simulink model "light_luminance"  (Simulink 10.0)
settings: Solver=FixedStepAuto  StartTime=0.0  StopTime=60  FixedStep=fixedStep  MaxStep=0.2  RelTol=1e-3
values from neighbouring files (symbols this model uses):
  L0Source1 = 1200    [lightModel.m]
  startLightSource = 0    [lightModel.m]
  timeLightSource = 20    [lightModel.m]
settings Model: Creator=lixuansong  LastModifiedBy=Ozgur Ozmen
settings DataIOCC: SaveFormat=Dataset  ReturnWorkspaceOutputs=on
settings OptimizationCC: LifeSpan=auto
settings DebuggingCC: UnderspecifiedInitializationDetection=Simplified  MergeDetectMultiDrivingBlocksExec=error  SFUnexpectedBacktrackingDiag=error  SFNoUnconditionalDefaultTransitionDiag=error  SFExecutionAtInitializationDiag=warning  ArithmeticOperatorsInVariantConditions=error
settings HardwareCC: ProdBitPerPointer=64  ProdBitPerSizeT=64  ProdBitPerPtrDiffT=64  ProdLargestAtomicFloat=Float  ProdIntDivRoundTo=Zero  ProdEndianess=LittleEndian  ProdWordSize=64  ProdHWDeviceType=Intel->x86-64 (Windows64)
settings ModelReferenceCC: PropagateSignalLabelsOutOfModel=on
settings SFSimCC: SimUseLocalCustomCode=on  CustomCodeUndefinedFunction=FilterOut
settings RTWCC: RTWUseLocalCustomCode=on
settings CodeAppCC: StateflowObjectComments=off
settings GRTTargetCC: TargetLangStandard=C99 (ISO)  CombineOutputUpdateFcns=on  GRTInterface=off
settings ConfigComp: CovMetricSettings=dwe  CovHtmlReporting=off  CovSaveCumulativeToWorkspaceVar=off  CovSaveSingleToWorkspaceVar=off

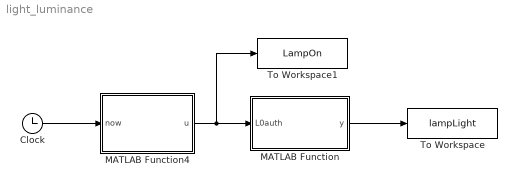
== system light_luminance ==
  Clock : Clock
  MATLAB Function : MATLAB Function  TreatAsAtomicUnit=on
  MATLAB Function4 : MATLAB Function  TreatAsAtomicUnit=on
  To Workspace : ToWorkspace  VariableName=lampLight  SampleTime=-1
  To Workspace1 : ToWorkspace  VariableName=LampOn  SampleTime=-1
  wires:
  MATLAB Function4/1(u) -> To Workspace1/1, MATLAB Function/1(L0auth)
  Clock/1 -> MATLAB Function4/1(now)
  MATLAB Function/1(y) -> To Workspace/1

== matlab function MATLAB Function ==
  data: L0auth input double; y output double; disLightSource parameter double
function y = calcLight(L0auth,disLightSource)

y=L0auth/(4*pi*disLightSource*disLightSource);

== matlab function MATLAB Function4 ==
  data: u output double; now input double; startLightSource parameter double; timeLightSource parameter double; L0Source1 parameter double
function u = controlLightSource(now,startLightSource,timeLightSource,L0Source1)
if now>=startLightSource && now<=startLightSource+timeLightSource
    u=L0Source1;
else
    u=0;
end
